simulink model "induction_machine"  (R2016a)
settings: Solver=VariableStepAuto  StartTime=0.0  StopTime=10.0  RelTol=1e-3
values from neighbouring files (symbols this model uses):
  Ibase_abc = 1/3*Sbase/Vbase_abc    [induction_machine_per_unit_bases.m]
  inv_TC = inv(TC)    [induction_machine_script.m]
  J = [ ... (first row only)    [induction_machine_script.m]
  J0 = [ ... (first row only)    [induction_machine_script.m]
  P = 6    [induction_machine_script.m]
  psi_rdq0_initial_condition = x0(4:6)    [induction_machine_script.m]
  psi_sdq0_initial_condition = x0(1:3)    [induction_machine_script.m]
  rr = rrfactor*0.0222    (= 0.0888)    [induction_machine_script.m]
  rs = rs +real(Z_line_pu)    [induction_machine_script.m]
  Tbase = Prated/(2/P*wbase)    [induction_machine_per_unit_bases.m]
  TC = [ ... (first row only)    [induction_machine_script.m]
  Vbase_abc = 1/sqrt(3)*Vrated    [induction_machine_per_unit_bases.m]
  wbase = 2*pi*frated    [induction_machine_per_unit_bases.m]
  Xa = 1/(1/XM + 1/Xls + 1/Xlr)    (= 0.0224977737592)    [induction_machine_script.m]
  Xlr = we_pu*Xlr    [induction_machine_equivalent_t.m]    (also in induction_machine_ic.m; induction_machine_script.m = 0.0322; induction_machine_ssop.m)
  Xls = we_pu*Xls    [induction_machine_equivalent_t.m]    (also in induction_machine_ic.m; induction_machine_script.m = Xls + imag(Z_line_pu); induction_machine_ssop.m)
settings Model: Creator=Seth Barger  LastModifiedBy=Seth Barger
settings OptimizationCC: DefaultParameterBehavior=Inlined
settings ModelReferenceCC: ModelReferenceNumInstancesAllowed=Single

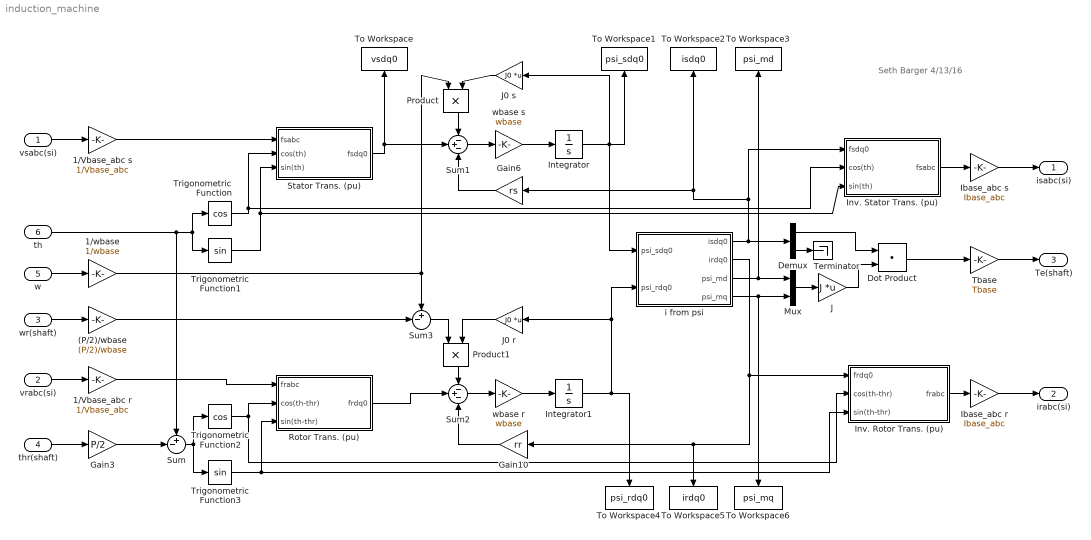
== system induction_machine ==
  note: Seth Barger
      | 4/13/16
  vsabc(si) : Inport
  vrabc(si) : Inport  Port=2
  wr(shaft) : Inport  Port=3
  thr(shaft) : Inport  Port=4
  w : Inport  Port=5
  th : Inport  Port=6
  (P/2)/wbase : Gain  Gain=(P/2)/wbase
  1/Vbase_abc r : Gain  Gain=1/Vbase_abc
  1/Vbase_abc s : Gain  Gain=1/Vbase_abc
  1/wbase : Gain  Gain=1/wbase
  Demux : Demux  Outputs=[2,1]
  Dot Product : DotProduct  InputSameDT=on  OutDataTypeStr=Inherit: Inherit via internal rule
  Gain10 : Gain  Gain=rr
  Gain3 : Gain  Gain=P/2
  Gain6 : Gain  Gain=rs
  Ibase_abc r : Gain  Gain=Ibase_abc
  Ibase_abc s : Gain  Gain=Ibase_abc
  Integrator : Integrator  InitialCondition=psi_sdq0_initial_condition
  Integrator1 : Integrator  InitialCondition=psi_rdq0_initial_condition
  Inv. Rotor Trans. (pu) : Subsystem
  Inv. Stator Trans. (pu) : Subsystem
  "J " : Gain  Gain=J  Multiplication=Matrix(K*u) (u vector)
  J0 r : Gain  Gain=J0  Multiplication=Matrix(K*u) (u vector)
  J0 s : Gain  Gain=J0  Multiplication=Matrix(K*u) (u vector)
  Mux : Mux  Inputs=2
  Product : Product
  Product1 : Product
  Rotor Trans. (pu) : Subsystem
  Stator Trans. (pu) : Subsystem
  Sum : Sum  Inputs=+-|
  Sum1 : Sum  Inputs=-+-
  Sum2 : Sum  Inputs=-+-
  Sum3 : Sum  Inputs=+-|
  Tbase : Gain  Gain=Tbase
  Terminator : Terminator
  To Workspace : ToWorkspace  VariableName=vsdq0  SampleTime=-1
  To Workspace1 : ToWorkspace  VariableName=psi_sdq0  SampleTime=-1
  To Workspace2 : ToWorkspace  VariableName=isdq0  SampleTime=-1
  To Workspace3 : ToWorkspace  VariableName=psi_md  SampleTime=-1
  To Workspace4 : ToWorkspace  VariableName=psi_rdq0  SampleTime=-1
  To Workspace5 : ToWorkspace  VariableName=irdq0  SampleTime=-1
  To Workspace6 : ToWorkspace  VariableName=psi_mq  SampleTime=-1
  Trigonometric Function : Trigonometry  Operator=cos
  Trigonometric Function1 : Trigonometry
  Trigonometric Function2 : Trigonometry  Operator=cos
  Trigonometric Function3 : Trigonometry
  i from psi : Subsystem
  wbase r : Gain  Gain=wbase
  wbase s : Gain  Gain=wbase
  isabc(si) : Outport
  irabc(si) : Outport  Port=2
  Te(shaft) : Outport  Port=3
  wires:
  vsabc(si)/1 -> 1/Vbase_abc s/1
  w/1 -> 1/wbase/1
  wr(shaft)/1 -> (P/2)/wbase/1
  vrabc(si)/1 -> 1/Vbase_abc r/1
  thr(shaft)/1 -> Gain3/1
  Gain3/1 -> Sum/2
  th/1 -> Sum/1, Trigonometric Function/1, Trigonometric Function1/1
  Sum/1 -> Trigonometric Function3/1, Trigonometric Function2/1
  1/Vbase_abc s/1 -> Stator Trans. (pu)/1(fsabc)
  Trigonometric Function/1 -> Inv. Stator Trans. (pu)/2(cos(th)), Stator Trans. (pu)/2(cos(th))
  Trigonometric Function1/1 -> Inv. Stator Trans. (pu)/3(sin(th)), Stator Trans. (pu)/3(sin(th))
  Stator Trans. (pu)/1(fsdq0) -> Sum1/2, To Workspace/1
  1/Vbase_abc r/1 -> Rotor Trans. (pu)/1(frabc)
  Trigonometric Function2/1 -> Inv. Rotor Trans. (pu)/2(cos(th-thr)), Rotor Trans. (pu)/2(cos(th-thr))
  Trigonometric Function3/1 -> Inv. Rotor Trans. (pu)/3(sin(th-thr)), Rotor Trans. (pu)/3(sin(th-thr))
  Product/1 -> Sum1/1
  Sum1/1 -> wbase s/1
  J0 s/1 -> Product/2
  Gain6/1 -> Sum1/3
  wbase s/1 -> Integrator/1
  Integrator/1 -> i from psi/1(psi_sdq0), To Workspace1/1, J0 s/1
  Rotor Trans. (pu)/1(frdq0) -> Sum2/2
  Product1/1 -> Sum2/1
  (P/2)/wbase/1 -> Sum3/2
  Sum3/1 -> Product1/1
  1/wbase/1 -> Product/1, Sum3/1
  J0 r/1 -> Product1/2
  Sum2/1 -> wbase r/1
  Gain10/1 -> Sum2/3
  wbase r/1 -> Integrator1/1
  Integrator1/1 -> To Workspace4/1, i from psi/2(psi_rdq0), J0 r/1
  i from psi/1(isdq0) -> Inv. Stator Trans. (pu)/1(fsdq0), Gain6/1, To Workspace2/1, Demux/1
  i from psi/3(psi_md) -> Mux/1, To Workspace3/1
  i from psi/2(irdq0) -> Inv. Rotor Trans. (pu)/1(frdq0), Gain10/1, To Workspace5/1
  i from psi/4(psi_mq) -> Mux/2, To Workspace6/1
  Inv. Stator Trans. (pu)/1(fsabc) -> Ibase_abc s/1
  Inv. Rotor Trans. (pu)/1(frabc) -> Ibase_abc r/1
  Ibase_abc r/1 -> irabc(si)/1
  Ibase_abc s/1 -> isabc(si)/1
  Demux/2 -> Terminator/1
  Mux/1 -> "J "/1
  Demux/1 -> Dot Product/1
  "J "/1 -> Dot Product/2
  Dot Product/1 -> Tbase/1
  Tbase/1 -> Te(shaft)/1

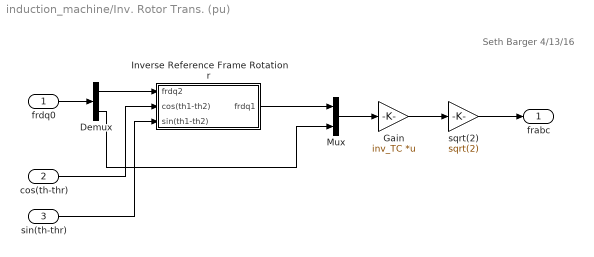
== system induction_machine/Inv. Rotor Trans. (pu) ==
  note: Seth Barger
      | 4/13/16
  frdq0 : Inport
  cos(th-thr) : Inport  Port=2
  sin(th-thr) : Inport  Port=3
  Demux : Demux  Outputs=[2,1]
  Gain : Gain  Gain=inv_TC  Multiplication=Matrix(K*u) (u vector)
  Inverse Reference Frame Rotation r : Subsystem
  Mux : Mux  Inputs=[2,1]
  sqrt(2) : Gain  Gain=sqrt(2)
  frabc : Outport
  wires:
  frdq0/1 -> Demux/1
  Demux/1 -> Inverse Reference Frame Rotation r/1(frdq2)
  Inverse Reference Frame Rotation r/1(frdq1) -> Mux/1
  Demux/2 -> Mux/2
  cos(th-thr)/1 -> Inverse Reference Frame Rotation r/2(cos(th1-th2))
  sin(th-thr)/1 -> Inverse Reference Frame Rotation r/3(sin(th1-th2))
  Mux/1 -> Gain/1
  Gain/1 -> sqrt(2)/1
  sqrt(2)/1 -> frabc/1

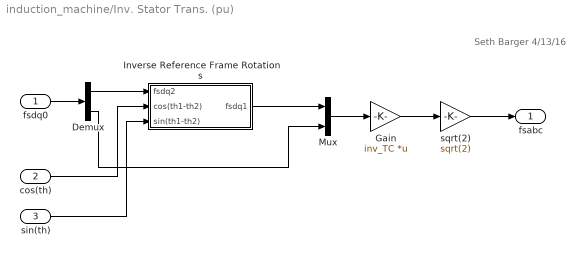
== system induction_machine/Inv. Stator Trans. (pu) ==
  note: Seth Barger
      | 4/13/16
  fsdq0 : Inport
  cos(th) : Inport  Port=2
  sin(th) : Inport  Port=3
  Demux : Demux  Outputs=[2,1]
  Gain : Gain  Gain=inv_TC  Multiplication=Matrix(K*u) (u vector)
  Inverse Reference Frame Rotation s : Subsystem
  Mux : Mux  Inputs=[2,1]
  sqrt(2) : Gain  Gain=sqrt(2)
  fsabc : Outport
  wires:
  fsdq0/1 -> Demux/1
  Demux/1 -> Inverse Reference Frame Rotation s/1(fsdq2)
  Inverse Reference Frame Rotation s/1(fsdq1) -> Mux/1
  Demux/2 -> Mux/2
  cos(th)/1 -> Inverse Reference Frame Rotation s/2(cos(th1-th2))
  sin(th)/1 -> Inverse Reference Frame Rotation s/3(sin(th1-th2))
  Mux/1 -> Gain/1
  Gain/1 -> sqrt(2)/1
  sqrt(2)/1 -> fsabc/1

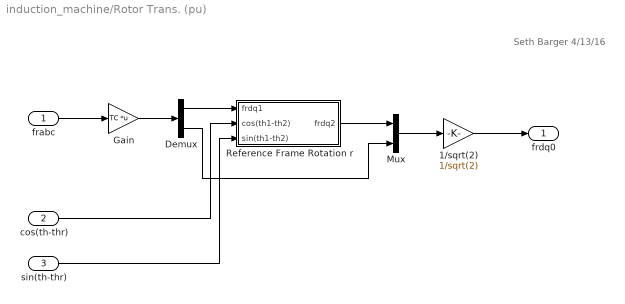
== system induction_machine/Rotor Trans. (pu) ==
  note: Seth Barger
      | 4/13/16
  frabc : Inport
  cos(th-thr) : Inport  Port=2
  sin(th-thr) : Inport  Port=3
  1/sqrt(2) : Gain  Gain=1/sqrt(2)
  Demux : Demux  Outputs=2
  Gain : Gain  Gain=TC  Multiplication=Matrix(K*u) (u vector)
  Mux : Mux  Inputs=[2,1]
  Reference Frame Rotation r : Subsystem
  frdq0 : Outport
  wires:
  frabc/1 -> Gain/1
  Gain/1 -> Demux/1
  Reference Frame Rotation r/1(frdq2) -> Mux/1
  Demux/2 -> Mux/2
  1/sqrt(2)/1 -> frdq0/1
  Mux/1 -> 1/sqrt(2)/1
  Demux/1 -> Reference Frame Rotation r/1(frdq1)
  cos(th-thr)/1 -> Reference Frame Rotation r/2(cos(th1-th2))
  sin(th-thr)/1 -> Reference Frame Rotation r/3(sin(th1-th2))

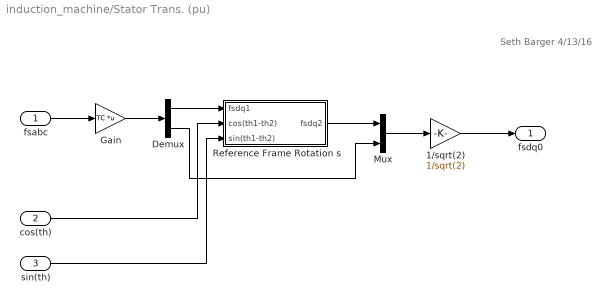
== system induction_machine/Stator Trans. (pu) ==
  note: Seth Barger
      | 4/13/16
  fsabc : Inport
  cos(th) : Inport  Port=2
  sin(th) : Inport  Port=3
  1/sqrt(2) : Gain  Gain=1/sqrt(2)
  Demux : Demux  Outputs=2
  Gain : Gain  Gain=TC  Multiplication=Matrix(K*u) (u vector)
  Mux : Mux  Inputs=[2,1]
  Reference Frame Rotation s : Subsystem
  fsdq0 : Outport
  wires:
  fsabc/1 -> Gain/1
  Gain/1 -> Demux/1
  Reference Frame Rotation s/1(fsdq2) -> Mux/1
  Demux/2 -> Mux/2
  1/sqrt(2)/1 -> fsdq0/1
  Mux/1 -> 1/sqrt(2)/1
  Demux/1 -> Reference Frame Rotation s/1(fsdq1)
  cos(th)/1 -> Reference Frame Rotation s/2(cos(th1-th2))
  sin(th)/1 -> Reference Frame Rotation s/3(sin(th1-th2))

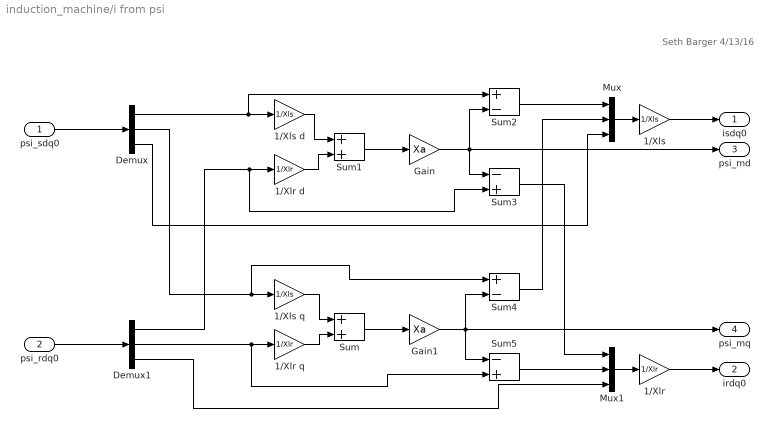
== system induction_machine/i from psi ==
  note: Seth Barger
      | 4/13/16
  psi_sdq0 : Inport
  psi_rdq0 : Inport  Port=2
  1/Xlr : Gain  Gain=1/Xlr
  1/Xlr d : Gain  Gain=1/Xlr
  1/Xlr q : Gain  Gain=1/Xlr
  1/Xls : Gain  Gain=1/Xls
  1/Xls d : Gain  Gain=1/Xls
  1/Xls q : Gain  Gain=1/Xls
  Demux : Demux  Outputs=3
  Demux1 : Demux  Outputs=3
  Gain : Gain  Gain=Xa
  Gain1 : Gain  Gain=Xa
  Mux : Mux  Inputs=3
  Mux1 : Mux  Inputs=3
  Sum : Sum
  Sum1 : Sum
  Sum2 : Sum  Inputs=+-
  Sum3 : Sum  Inputs=-+
  Sum4 : Sum  Inputs=+-
  Sum5 : Sum  Inputs=-+
  isdq0 : Outport
  irdq0 : Outport  Port=2
  psi_md : Outport  Port=3
  psi_mq : Outport  Port=4
  wires:
  psi_sdq0/1 -> Demux/1
  psi_rdq0/1 -> Demux1/1
  Demux/1 -> Sum2/1, 1/Xls d/1
  Demux1/1 -> Sum3/2, 1/Xlr d/1
  Demux1/2 -> Sum5/2, 1/Xlr q/1
  Demux/2 -> Sum4/1, 1/Xls q/1
  1/Xls q/1 -> Sum/1
  1/Xlr q/1 -> Sum/2
  1/Xls d/1 -> Sum1/1
  1/Xlr d/1 -> Sum1/2
  Sum/1 -> Gain1/1
  Sum1/1 -> Gain/1
  Gain1/1 -> Sum4/2, psi_mq/1, Sum5/1
  Gain/1 -> Sum3/1, Sum2/2, psi_md/1
  Sum2/1 -> Mux/1
  Sum5/1 -> Mux1/2
  Sum3/1 -> Mux1/1
  Sum4/1 -> Mux/2
  Demux/3 -> Mux/3
  Demux1/3 -> Mux1/3
  Mux1/1 -> 1/Xlr/1
  1/Xlr/1 -> irdq0/1
  1/Xls/1 -> isdq0/1
  Mux/1 -> 1/Xls/1

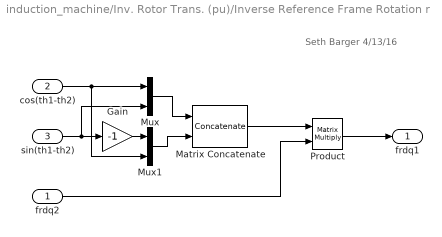
== system induction_machine/Inv. Rotor Trans. (pu)/Inverse Reference Frame Rotation r ==
  note: Seth Barger
      | 4/13/16
  frdq2 : Inport
  cos(th1-th2) : Inport  Port=2
  sin(th1-th2) : Inport  Port=3
  Gain : Gain  Gain=-1
  Matrix Concatenate : Concatenate  Mode=Multidimensional array  ConcatenateDimension=2
  Mux : Mux  Inputs=2
  Mux1 : Mux  Inputs=2
  Product : Product  Multiplication=Matrix(*)
  frdq1 : Outport
  wires:
  cos(th1-th2)/1 -> Mux1/2, Mux/1
  sin(th1-th2)/1 -> Gain/1, Mux/2
  Gain/1 -> Mux1/1
  Mux1/1 -> Matrix Concatenate/2
  Mux/1 -> Matrix Concatenate/1
  Matrix Concatenate/1 -> Product/1
  frdq2/1 -> Product/2
  Product/1 -> frdq1/1

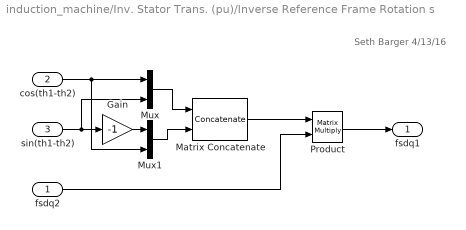
== system induction_machine/Inv. Stator Trans. (pu)/Inverse Reference Frame Rotation s ==
  note: Seth Barger
      | 4/13/16
  fsdq2 : Inport
  cos(th1-th2) : Inport  Port=2
  sin(th1-th2) : Inport  Port=3
  Gain : Gain  Gain=-1
  Matrix Concatenate : Concatenate  Mode=Multidimensional array  ConcatenateDimension=2
  Mux : Mux  Inputs=2
  Mux1 : Mux  Inputs=2
  Product : Product  Multiplication=Matrix(*)
  fsdq1 : Outport
  wires:
  cos(th1-th2)/1 -> Mux1/2, Mux/1
  sin(th1-th2)/1 -> Gain/1, Mux/2
  Gain/1 -> Mux1/1
  Mux1/1 -> Matrix Concatenate/2
  Mux/1 -> Matrix Concatenate/1
  Matrix Concatenate/1 -> Product/1
  fsdq2/1 -> Product/2
  Product/1 -> fsdq1/1

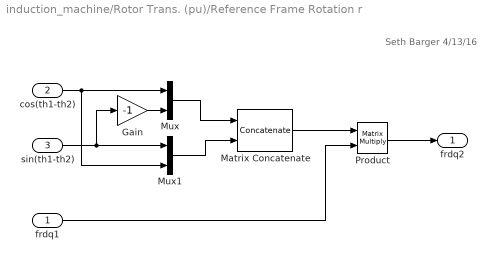
== system induction_machine/Rotor Trans. (pu)/Reference Frame Rotation r ==
  note: Seth Barger
      | 4/13/16
  frdq1 : Inport
  cos(th1-th2) : Inport  Port=2
  sin(th1-th2) : Inport  Port=3
  Gain : Gain  Gain=-1
  Matrix Concatenate : Concatenate  Mode=Multidimensional array  ConcatenateDimension=2
  Mux : Mux  Inputs=2
  Mux1 : Mux  Inputs=2
  Product : Product  Multiplication=Matrix(*)
  frdq2 : Outport
  wires:
  sin(th1-th2)/1 -> Gain/1, Mux1/1
  cos(th1-th2)/1 -> Mux/1, Mux1/2
  Gain/1 -> Mux/2
  Mux/1 -> Matrix Concatenate/1
  Mux1/1 -> Matrix Concatenate/2
  Product/1 -> frdq2/1
  Matrix Concatenate/1 -> Product/1
  frdq1/1 -> Product/2

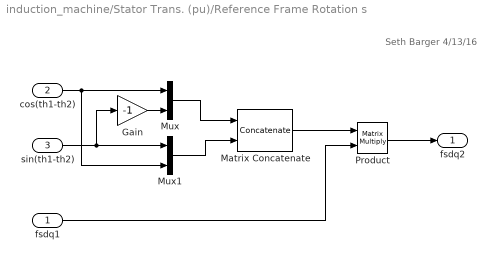
== system induction_machine/Stator Trans. (pu)/Reference Frame Rotation s ==
  note: Seth Barger
      | 4/13/16
  fsdq1 : Inport
  cos(th1-th2) : Inport  Port=2
  sin(th1-th2) : Inport  Port=3
  Gain : Gain  Gain=-1
  Matrix Concatenate : Concatenate  Mode=Multidimensional array  ConcatenateDimension=2
  Mux : Mux  Inputs=2
  Mux1 : Mux  Inputs=2
  Product : Product  Multiplication=Matrix(*)
  fsdq2 : Outport
  wires:
  sin(th1-th2)/1 -> Gain/1, Mux1/1
  cos(th1-th2)/1 -> Mux/1, Mux1/2
  Gain/1 -> Mux/2
  Mux/1 -> Matrix Concatenate/1
  Mux1/1 -> Matrix Concatenate/2
  Product/1 -> fsdq2/1
  Matrix Concatenate/1 -> Product/1
  fsdq1/1 -> Product/2
